simulink model "DynamicModelSteadyState"  (R2018a)
settings: Solver=FixedStepAuto  StartTime=0.0  StopTime=10  RelTol=1e-3
model workspace (MAT data in the model file):
  Iz = 0.0452
  cf = 70
  cr = 70
  k1 = 1
  k2 = 0.5673
  k3 = 2.6383
  k4 = 0.4975
  lf = 0.16002
  lr = 0.16002
  m = 3
libraries: simulink_extras x2, templibrary x1
settings Model: PacingRate=0.100000  Creator=aswerdlow  LastModifiedBy=aswer
settings SolverCC: AlgebraicLoopSolver=LineSearch
settings OptimizationCC: DefaultParameterBehavior=Inlined  UseDivisionForNetSlopeComputation=on  UseFloatMulNetSlope=on  InlineInvariantSignals=on  PassReuseOutputArgsAs=Individual arguments  ZeroExternalMemoryAtStartup=off  ZeroInternalMemoryAtStartup=off  NoFixptDivByZeroProtection=on  EfficientFloat2IntCast=on  LifeSpan=1  OptimizeBlockOrder=speed  DifferentSizesBufferReuse=on
settings DebuggingCC: ParameterTunabilityLossMsg=error
settings HardwareCC: ProdLongLongMode=on
settings SFSimCC: MATLABDynamicMemAlloc=off
settings RTWCC: SystemTargetFile=ert.tlc  TemplateMakefile=ert_default_tmf  GenerateReport=on  IncludeHyperlinkInReport=on  LaunchReport=on  TargetLang=C++  GenerateTraceInfo=on  GenerateTraceReport=on  GenerateTraceReportSl=on  GenerateTraceReportSf=on  GenerateTraceReportEml=on
settings CodeAppCC: ForceParamTrailComments=on  IgnoreCustomStorageClasses=off  OperatorAnnotations=on  SimulinkDataObjDesc=on  SFDataObjDesc=on  CustomSymbolStrGlobalVar=rt$N$M  CustomSymbolStrType=$N$M  CustomSymbolStrFcn=$N$M$F  CustomSymbolStrMacro=$N$M  InsertBlockDesc=on
settings ERTTargetCC: TargetLangStandard=C++03 (ISO)  GenerateSampleERTMain=on  IncludeMdlTerminateFcn=off  CombineSignalStateStructs=on  SupportAbsoluteTime=off  MultiInstanceERTCode=on  CodeInterfacePackaging=C++ class  SupportComplex=off  SupportContinuousTime=on  SupportNonInlinedSFcns=on  InlinedParameterPlacement=NonHierarchical  RootIOFormat=Structure reference  ERTCustomFileTemplate=example_file_process.tlc  ERTFilePackagingFormat=CompactWithDataFile

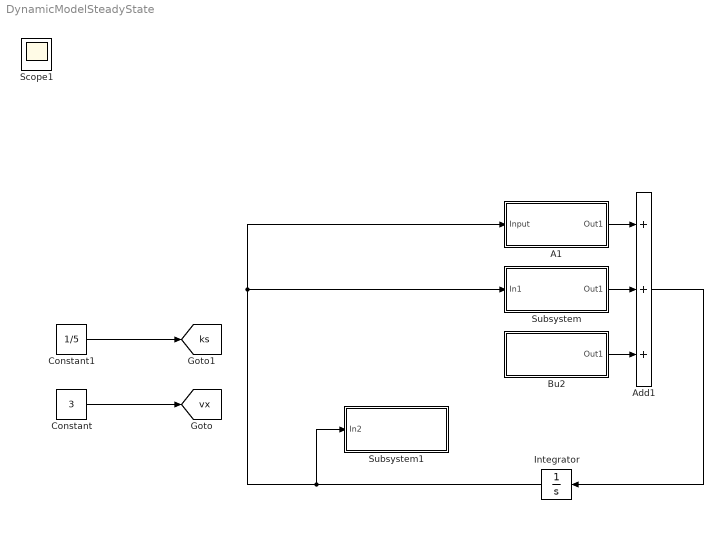
== system DynamicModelSteadyState ==
  A1 : Subsystem
  Add1 : Sum  Inputs=+++
  Bu2 : Subsystem
  Constant : Constant  Value=3
  Constant1 : Constant  Value=1/5
  Integrator : Integrator
  Subsystem : Subsystem
  Subsystem1 : Subsystem
  Scope1 : Scope
  tag scope: ks=global, vx=global
  wires:
  Add1/1 -> Integrator/1
  Integrator/1 -> Subsystem1/1(In2), A1/1(Input), Subsystem/1(In1)
  Subsystem/1(Out1) -> Add1/2
  A1/1(Out1) -> Add1/1
  Bu2/1(Out1) -> Add1/3
  Constant/1 -> [vx]
  Constant1/1 -> [ks]

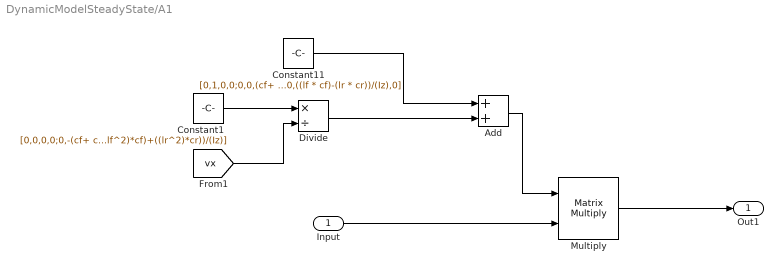
== system DynamicModelSteadyState/A1 ==
  Input : Inport
  Add : Sum
  Constant1 : Constant  Value=[0,0,0,0;0,-(cf+ cr)/(m),0,(lr * cr)-(lf * cf)/(m);0,0,0,0;0,((lr * cr)-(lf * cf))/(Iz),0,-(((lf^2)*cf)+((lr^2)*cr))/(Iz)]  VectorParams1D=off
  Constant11 : Constant  Value=[0,1,0,0;0,0,(cf+ cr)/(m),0;0,0,0,1;0,0,((lf * cf)-(lr * cr))/(Iz),0]  VectorParams1D=off
  Divide : Product  Inputs=*/
  Multiply : Product  Multiplication=Matrix(*)
  Out1 : Outport
  wires:
  [vx] -> Divide/2
  Constant11/1 -> Add/1
  Constant1/1 -> Divide/1
  Divide/1 -> Add/2
  Add/1 -> Multiply/1
  Input/1 -> Multiply/2
  Multiply/1 -> Out1/1

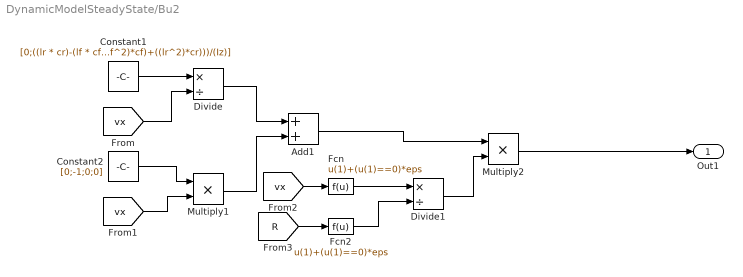
== system DynamicModelSteadyState/Bu2 ==
  Add1 : Sum
  Constant1 : Constant  Value=[0;((lr * cr)-(lf * cf))/m;0;(-(((lf^2)*cf)+((lr^2)*cr)))/(Iz)]  VectorParams1D=off
  Constant2 : Constant  Value=[0;-1;0;0]
  Divide : Product  Inputs=*/
  Divide1 : Product  Inputs=*/
  Fcn : Fcn  Expr=u(1)+(u(1)==0)*eps
  Fcn2 : Fcn  Expr=u(1)+(u(1)==0)*eps
  Multiply1 : Product
  Multiply2 : Product
  Out1 : Outport
  wires:
  Multiply2/1 -> Out1/1
  Constant1/1 -> Divide/1
  [vx] -> Divide/2
  Constant2/1 -> Multiply1/1
  [vx] -> Multiply1/2
  Divide/1 -> Add1/1
  Multiply1/1 -> Add1/2
  Add1/1 -> Multiply2/1
  [vx] -> Fcn/1
  [R] -> Fcn2/1
  Divide1/1 -> Multiply2/2
  Fcn/1 -> Divide1/1
  Fcn2/1 -> Divide1/2

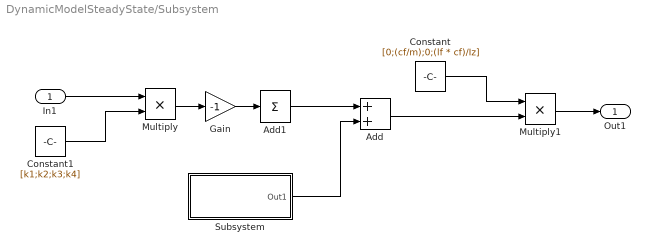
== system DynamicModelSteadyState/Subsystem ==
  In1 : Inport
  Add : Sum
  Add1 : Sum  Inputs=+
  Constant : Constant  Value=[0;(cf/m);0;(lf * cf)/Iz]
  Constant1 : Constant  Value=[k1;k2;k3;k4]
  Gain : Gain  Gain=-1
  Multiply : Product
  Multiply1 : Product
  Subsystem : Subsystem
  Out1 : Outport
  wires:
  In1/1 -> Multiply/1
  Constant1/1 -> Multiply/2
  Multiply/1 -> Gain/1
  Gain/1 -> Add1/1
  Subsystem/1(Out1) -> Add/2
  Add/1 -> Multiply1/2
  Constant/1 -> Multiply1/1
  Multiply1/1 -> Out1/1
  Add1/1 -> Add/1

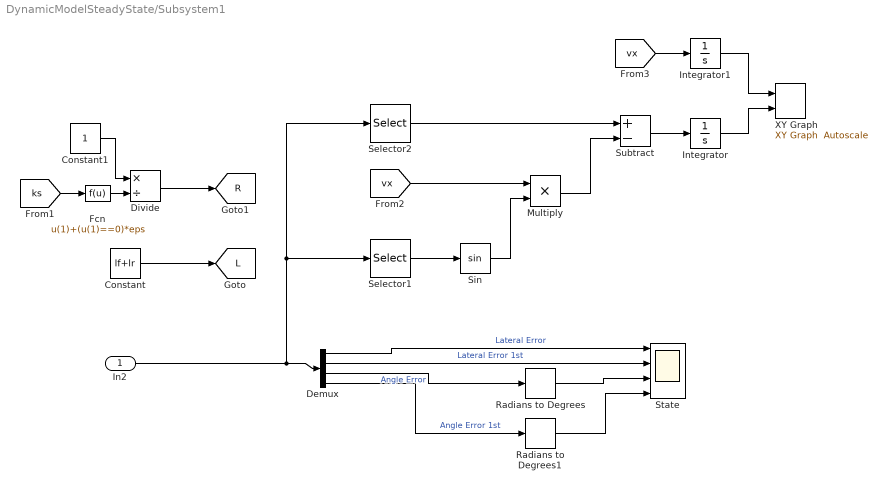
== system DynamicModelSteadyState/Subsystem1 ==
  In2 : Inport
  Constant : Constant  Value=lf+lr
  Constant1 : Constant
  Demux : Demux
  Divide : Product  Inputs=*/
  Fcn : Fcn  Expr=u(1)+(u(1)==0)*eps
  Integrator : Integrator
  Integrator1 : Integrator
  Multiply : Product
  Radians to Degrees : simulink_extras/Transformations/Radians to Degrees
  Radians to Degrees1 : simulink_extras/Transformations/Radians to Degrees
  Selector1 : Selector  InputPortWidth=4  IndexOptions=Index vector (dialog)  Indices=3  OutputSizes=1
  Selector2 : Selector  InputPortWidth=4  IndexOptions=Index vector (dialog)  Indices=2  OutputSizes=1
  Sin : Trigonometry
  State : Scope  NumInputPorts=4
  Subtract : Sum  Inputs=+-
  XY Graph : templibrary/XY Graph  Autoscale  xmin=-1  xmax=1  ymin=-1  ymax=1  st=-1
  tag scope: L=global, R=global
  wires:
  Constant/1 -> [L]
  In2/1 -> Selector2/1, Selector1/1, Demux/1
  Divide/1 -> [R]
  [ks] -> Fcn/1
  Constant1/1 -> Divide/1
  Fcn/1 -> Divide/2
  Sin/1 -> Multiply/2
  [vx] -> Integrator1/1
  Multiply/1 -> Subtract/2
  [vx] -> Multiply/1
  Selector1/1 -> Sin/1
  Selector2/1 -> Subtract/1
  Integrator/1 -> XY Graph/2
  Subtract/1 -> Integrator/1
  Integrator1/1 -> XY Graph/1
  Demux/1 -> State/1  "Lateral Error"
  Demux/2 -> State/2  "Lateral Error 1st"
  Demux/3 -> Radians to Degrees/1  "Angle Error"
  Demux/4 -> Radians to Degrees1/1  "Angle Error 1st"
  Radians to Degrees/1 -> State/3
  Radians to Degrees1/1 -> State/4

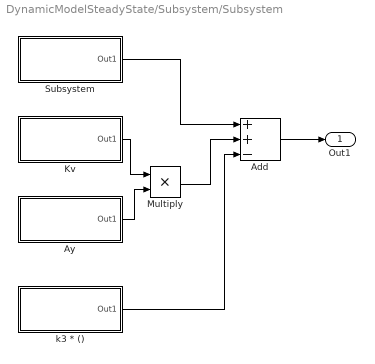
== system DynamicModelSteadyState/Subsystem/Subsystem ==
  Add : Sum  Inputs=++-
  Ay : Subsystem
  Kv : Subsystem
  Multiply : Product
  Subsystem : Subsystem
  k3 * () : Subsystem
  Out1 : Outport
  wires:
  Kv/1(Out1) -> Multiply/1
  Ay/1(Out1) -> Multiply/2
  Multiply/1 -> Add/2
  Add/1 -> Out1/1
  k3 * ()/1(Out1) -> Add/3
  Subsystem/1(Out1) -> Add/1

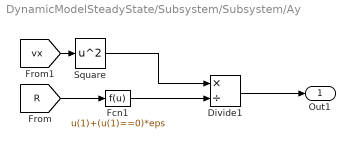
== system DynamicModelSteadyState/Subsystem/Subsystem/Ay ==
  Divide1 : Product  Inputs=*/
  Fcn1 : Fcn  Expr=u(1)+(u(1)==0)*eps
  Square : Math  Operator=square  SaturateOnIntegerOverflow=on
  Out1 : Outport
  wires:
  [R] -> Fcn1/1
  Square/1 -> Divide1/1
  Fcn1/1 -> Divide1/2
  [vx] -> Square/1
  Divide1/1 -> Out1/1

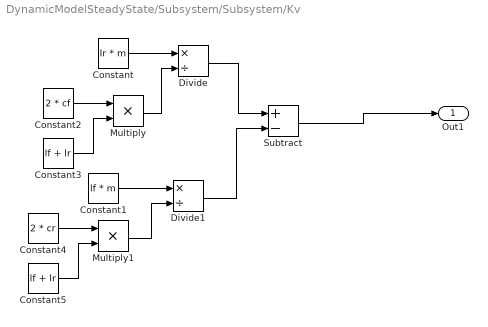
== system DynamicModelSteadyState/Subsystem/Subsystem/Kv ==
  Constant : Constant  Value=lr * m
  Constant1 : Constant  Value=lf * m
  Constant2 : Constant  Value=2 * cf
  Constant3 : Constant  Value=lf + lr
  Constant4 : Constant  Value=2 * cr
  Constant5 : Constant  Value=lf + lr
  Divide : Product  Inputs=*/
  Divide1 : Product  Inputs=*/
  Multiply : Product
  Multiply1 : Product
  Subtract : Sum  Inputs=+-
  Out1 : Outport
  wires:
  Divide/1 -> Subtract/1
  Divide1/1 -> Subtract/2
  Constant/1 -> Divide/1
  Constant1/1 -> Divide1/1
  Constant2/1 -> Multiply/1
  Constant3/1 -> Multiply/2
  Multiply/1 -> Divide/2
  Constant5/1 -> Multiply1/2
  Constant4/1 -> Multiply1/1
  Multiply1/1 -> Divide1/2
  Subtract/1 -> Out1/1

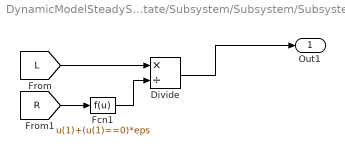
== system DynamicModelSteadyState/Subsystem/Subsystem/Subsystem ==
  Divide : Product  Inputs=*/
  Fcn1 : Fcn  Expr=u(1)+(u(1)==0)*eps
  Out1 : Outport
  wires:
  [L] -> Divide/1
  Divide/1 -> Out1/1
  [R] -> Fcn1/1
  Fcn1/1 -> Divide/2

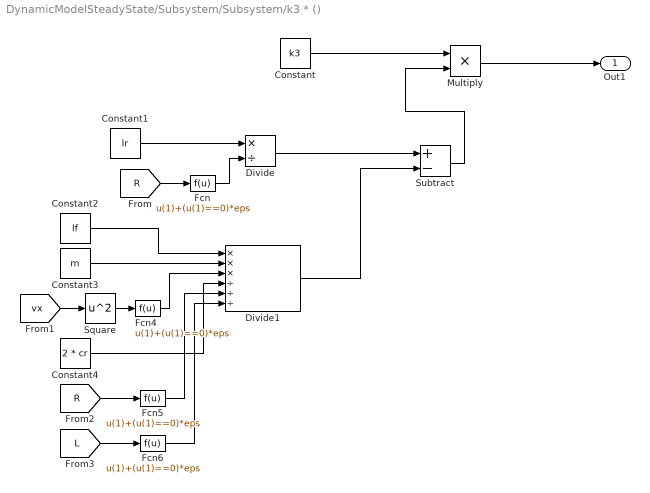
== system DynamicModelSteadyState/Subsystem/Subsystem/k3 * () ==
  Constant : Constant  Value=k3
  Constant1 : Constant  Value=lr
  Constant2 : Constant  Value=lf
  Constant3 : Constant  Value=m
  Constant4 : Constant  Value=2 * cr
  Divide : Product  Inputs=*/
  Divide1 : Product  Inputs=***///
  Fcn{,4..6} (4 alike) : Fcn  Expr=u(1)+(u(1)==0)*eps
  Multiply : Product
  Square : Math  Operator=square  SaturateOnIntegerOverflow=on
  Subtract : Sum  Inputs=+-
  Out1 : Outport
  wires:
  Constant/1 -> Multiply/1
  Multiply/1 -> Out1/1
  Divide/1 -> Subtract/1
  Constant1/1 -> Divide/1
  Divide1/1 -> Subtract/2
  Constant2/1 -> Divide1/1
  Constant3/1 -> Divide1/2
  [vx] -> Square/1
  Square/1 -> Fcn4/1
  Constant4/1 -> Divide1/4
  [R] -> Fcn5/1
  [L] -> Fcn6/1
  Subtract/1 -> Multiply/2
  [R] -> Fcn/1
  Fcn6/1 -> Divide1/6
  Fcn5/1 -> Divide1/5
  Fcn4/1 -> Divide1/3
  Fcn/1 -> Divide/2
